simulink model "Simulator_3D2"  (R2018a)
settings: Solver=ode4  StartTime=0.0  StopTime=60  FixedStep=T  RelTol=1e-3
undefined symbols (not defined in the file): A_w, A_w2, epsilon_w, epsilon_w2, k_w, k_w2, Lc_0, omega_w, omega_w2, T, w_dir, w_dir2, zu_bar
libraries: vrlib x132
(part 1 of 6)
settings Model: Creator=Ahmad  LastModifiedBy=Ahmad

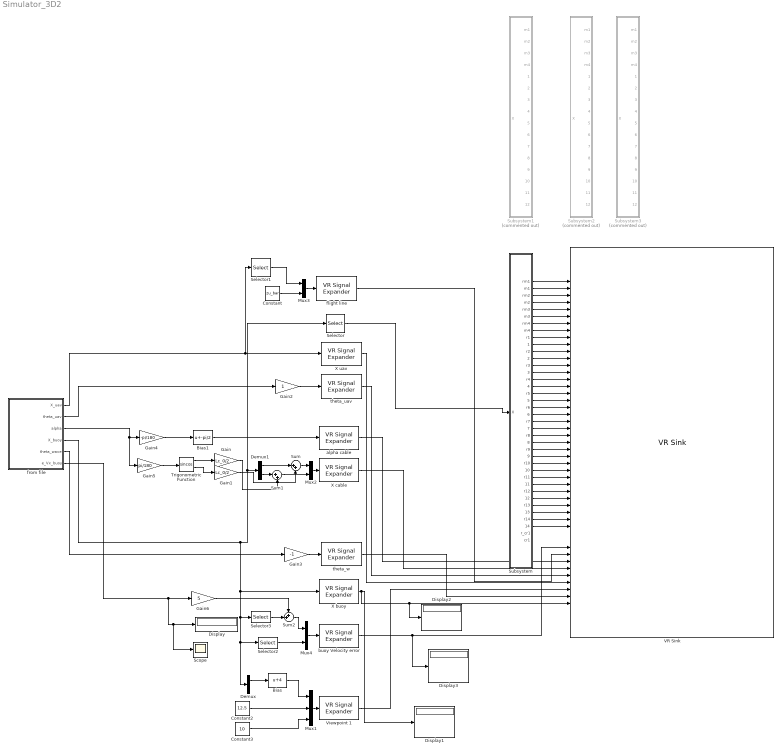
== system Simulator_3D2 ==
  Bias : Bias  Bias=4
  Bias1 : Bias  Bias=-pi/2
  Constant : Constant  Value=zu_bar
  Constant2 : Constant  Value=12.5
  Constant3 : Constant  Value=10
  Demux : Demux  Outputs=2
  Demux1 : Demux  Outputs=2
  Display{,1..3} (4 alike) : Display
  Gain : Gain  Gain=Lc_0/2
  Gain1 : Gain  Gain=Lc_0/2
  Gain2 : Gain
  Gain3 : Gain  Gain=-1
  Gain4 : Gain  Gain=-pi/180
  Gain5 : Gain  Gain=pi/180
  Gain6 : Gain  Gain=5
  Mux1 : Mux  Inputs=3
  Mux2 : Mux  Inputs=2
  Mux3 : Mux  Inputs=2
  Mux4 : Mux  Inputs=2
  Scope : Scope
  Selector : Selector  InputPortWidth=2  IndexOptions=Index vector (dialog)  Indices=[1]  OutputSizes=1
  Selector1 : Selector  InputPortWidth=2  IndexOptions=Index vector (dialog)  Indices=[1]  OutputSizes=1
  Selector2 : Selector  InputPortWidth=2  IndexOptions=Index vector (dialog)  Indices=2  OutputSizes=1
  Selector3 : Selector  InputPortWidth=2  IndexOptions=Index vector (dialog)  Indices=1  OutputSizes=1
  Subsystem : Subsystem
  Subsystem1 : Subsystem  Commented=on
  Subsystem2 : Subsystem  Commented=on
  Subsystem3 : Subsystem  Commented=on
  Sum : Sum  Inputs=|++
  Sum1 : Sum  Inputs=|++
  Sum2 : Sum  Inputs=++|
  Trigonometric Function : Trigonometry  Operator=sincos
  VR Sink : vrlib/VR Sink  InstantiateOnLoad=on  SampleTime=T  ViewEnable=on  RemoteChange=off  RemoteView=off  FieldsWritten=wave_m1.rotation.4.1.1.double#wave_m1.translation.3.1.1.double#wave_m2.rotation.4.1.1.double#wave_m2.translation.3.1.1.double#wave_m3.rotation.4.1.1.double#wave_m3.translation.3.1.1.double#wave_m4.rotation.4.1.1.double#wave_m4.translation.3.1.1.double#wave_1.rotation.4.1.1.double#wave_1.translation.3.1.1.double#wave_2.rotation.4.1.1.double#wave_2.translation.3.1.1.double#wave_3.rotation.4.1.1.double#wave_3.translation.3.1.1.double#wave_4.rotation.4.1.1.double#wave_4.translation.3.1.1.double#wave_5.rotation.4.1.1.double#wave_5.translation.3.1.1.double#wave_6.rotation.4.1.1.double#wave_6.translation.3.1.1.double#wave_7.rotation.4.1.1.double#wave_7.translation.3.1.1.double#wave_8.rotation.4.1.1.double#wave_8.translation.3.1.1.double#wave_9.rotation.4.1.1.double#wave_9.translation.3.1.1.double#wave_10.rotation.4.1.1.double#wave_10.translation.3.1.1.double#wave_11.rotation.4.1.1.double#wave_11.translation.3.1.1.double#wave_12.rotation.4.1.1.double#wave_12.translation.3.1.1.double#wave_13.rotation.4.1.1.double#wave_13.translation.3.1.1.double#wave_14.rotation.4.1.1.double#wave_14.translation.3.1.1.double#crest_1.rotation.4.1.1.double#crest_1.translation.3.1.1.double#V_ref.translation.3.1.1.double#flight_line.translation.3.1.1.double#cable.rotation.4.1.1.double#cable.translation.3.1.1.double#UAV2.rotation.4.1.1.double#UAV2.translation.3.1.1.double#Viewpoint_1_uav.position.3.1.1.double#Buoy.rotation.4.1.1.double#Buoy.translation.3.1.1.double  WorldFileName=Scene_v2.wrl  AutoView=off  VideoDimensions=[]  AllowVariableSize=off  FigureProperties="{'Position', 'Name', 'Viewpoint', 'CameraBound', 'CameraDirection', 'CameraPosition', 'CameraUpVector', 'ZoomFactor', 'Antialiasing', 'Headlight', 'Lighting', 'NavPanel', 'Sound', 'StatusBar', 'Stereo3D', 'Stereo3DCameraOffset', 'Stereo3DHIT', 'ToolBar', 'Textures', 'Transparency', 'Triad', 'Wireframe', 'NavZones', 'NavMode', 'NavSpeed', 'CaptureFileFormat', 'CaptureFileName', 'Record2DCompressMethod', 'Record2DCompressQuality', 'Record2D', 'Record2DFileName', 'Record2DFPS'; [1.8800000000000000e+02   1.7400000000000000e+02   5.7600000000000000e+02   3.5000000000000000e+02], '', '_untitled_1', 'on', [0.0000000000000000e+00   0.0000000000000000e+00  -1.0000000000000000e+00], [0.0000000000000000e+00   0.0000000000000000e+00   0.0000000000000000e+00], [0.0000000000000000e+00   1.0000000000000000e+00   0.0000000000000000e+00], [1.0000000000000000e+00], 'on', 'on', 'on', 'halfbar', 'on', 'on', 'off', [1.0000000149011612e-01], [0.0000000000000000e+00], 'on', 'on', 'on', 'none', 'off', 'off', 'fly', 'normal', 'png', '%f_anim_%n.png', 'auto', [1.0000000000000000e+02], 'on', '%f_anim_%n.avi', 'auto'}"
      settings: SourceProductBaseCode=VR
  Viewpoint 1 : vrlib/VR Signal Expander  outwidth=3  outidx=[1 2 3]
      settings: SourceProductName=Simulink 3D Animation  SourceProductBaseCode=VR
  X buoy : vrlib/VR Signal Expander  outwidth=3  outidx=[1 2]
      settings: SourceProductName=Simulink 3D Animation  SourceProductBaseCode=VR
  X cable : vrlib/VR Signal Expander  outwidth=3  outidx=[1 2]
      settings: SourceProductName=Simulink 3D Animation  SourceProductBaseCode=VR
  X uav : vrlib/VR Signal Expander  outwidth=3  outidx=[1 2]
      settings: SourceProductName=Simulink 3D Animation  SourceProductBaseCode=VR
  alpha cable : vrlib/VR Signal Expander  outwidth=4  outidx=[4]
      settings: SourceProductName=Simulink 3D Animation  SourceProductBaseCode=VR
  buoy Velocity error : vrlib/VR Signal Expander  outwidth=3  outidx=[1 2]
      settings: SourceProductName=Simulink 3D Animation  SourceProductBaseCode=VR
  flight line : vrlib/VR Signal Expander  outwidth=3  outidx=[1 2]
      settings: SourceProductName=Simulink 3D Animation  SourceProductBaseCode=VR
  from file : Subsystem
  theta_uav : vrlib/VR Signal Expander  outwidth=4  outidx=[4]
      settings: SourceProductName=Simulink 3D Animation  SourceProductBaseCode=VR
  theta_w : vrlib/VR Signal Expander  outwidth=4  outidx=[4]
      settings: SourceProductName=Simulink 3D Animation  SourceProductBaseCode=VR
  wires:
  X buoy/1 -> Display1/1, Display2/1, VR Sink/47
  Mux1/1 -> Viewpoint 1/1
  Demux/1 -> Bias/1
  Constant2/1 -> Mux1/2
  Constant3/1 -> Mux1/3
  Bias/1 -> Mux1/1
  Trigonometric Function/1 -> Gain/1
  Trigonometric Function/2 -> Gain1/1
  Demux1/1 -> Sum/1
  Mux2/1 -> X cable/1
  Sum/1 -> Mux2/1
  Demux1/2 -> Sum1/1
  Sum1/1 -> Mux2/2
  Gain1/1 -> Sum/2
  Gain/1 -> Sum1/2
  Gain2/1 -> theta_uav/1
  Gain3/1 -> theta_w/1
  Gain4/1 -> Bias1/1
  Gain5/1 -> Trigonometric Function/1
  Bias1/1 -> alpha cable/1
  Selector/1 -> Subsystem/1(X)
  Selector1/1 -> Mux3/1
  Mux3/1 -> flight line/1
  Constant/1 -> Mux3/2
  from file/3(alpha) -> Gain5/1, Gain4/1
  from file/1(X_uav) -> Selector1/1, X uav/1
  from file/4(X_buoy) -> Demux1/1, Selector/1, X buoy/1, Selector2/1, Demux/1, Selector3/1
  from file/2(theta_uav) -> Gain2/1
  from file/5(theta_wave) -> Gain3/1
  Subsystem/1(rm1) -> VR Sink/1
  Subsystem/2(m1) -> VR Sink/2
  Subsystem/3(rm2) -> VR Sink/3
  Subsystem/4(m2) -> VR Sink/4
  Subsystem/5(rm3) -> VR Sink/5
  Subsystem/6(m3) -> VR Sink/6
  Subsystem/7(rm4) -> VR Sink/7
  Subsystem/8(m4) -> VR Sink/8
  Subsystem/9(r1) -> VR Sink/9
  Subsystem/10(1) -> VR Sink/10
  Subsystem/11(r2) -> VR Sink/11
  Subsystem/12(2) -> VR Sink/12
  Subsystem/13(r3) -> VR Sink/13
  Subsystem/14(3) -> VR Sink/14
  Subsystem/15(r4) -> VR Sink/15
  Subsystem/16(4) -> VR Sink/16
  Subsystem/17(r5) -> VR Sink/17
  Subsystem/18(5) -> VR Sink/18
  Subsystem/19(r6) -> VR Sink/19
  Subsystem/20(6) -> VR Sink/20
  Subsystem/21(r7) -> VR Sink/21
  Subsystem/22(7) -> VR Sink/22
  Subsystem/23(r8) -> VR Sink/23
  Subsystem/24(8) -> VR Sink/24
  Subsystem/25(r9) -> VR Sink/25
  Subsystem/26(9) -> VR Sink/26
  Subsystem/27(r10) -> VR Sink/27
  Subsystem/28(10) -> VR Sink/28
  Subsystem/29(r11) -> VR Sink/29
  Subsystem/30(11) -> VR Sink/30
  Subsystem/31(r12) -> VR Sink/31
  Subsystem/32(12) -> VR Sink/32
  Subsystem/33(r13) -> VR Sink/33
  Subsystem/34(13) -> VR Sink/34
  Subsystem/35(r14) -> VR Sink/35
  Subsystem/36(14) -> VR Sink/36
  ? -> VR Sink/37
  ? -> VR Sink/38
  flight line/1 -> VR Sink/40
  alpha cable/1 -> VR Sink/41
  X cable/1 -> VR Sink/42
  theta_uav/1 -> VR Sink/43
  X uav/1 -> VR Sink/44
  Viewpoint 1/1 -> VR Sink/45
  theta_w/1 -> VR Sink/46
  Mux4/1 -> buoy Velocity error/1
  Selector2/1 -> Mux4/2
  Sum2/1 -> Mux4/1
  Selector3/1 -> Sum2/2
  from file/6(e_Vx_buoy) -> Scope/1, Display/1, Gain6/1
  Gain6/1 -> Sum2/1
  buoy Velocity error/1 -> Display3/1, VR Sink/39

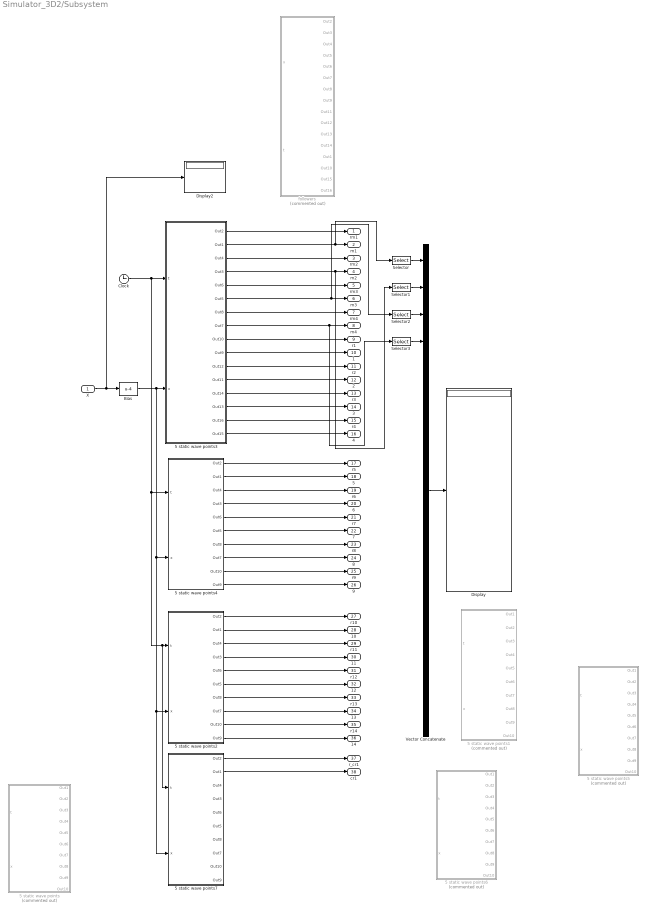
== system Simulator_3D2/Subsystem ==
  X : Inport
  5 static wave points : Subsystem  Commented=on
  5 static wave points1 : Subsystem  Commented=on
  5 static wave points2 : Subsystem
  5 static wave points3 : Subsystem
  5 static wave points4 : Subsystem
  5 static wave points5 : Subsystem  Commented=on
  5 static wave points6 : Subsystem  Commented=on
  5 static wave points7 : Subsystem
  Bias : Bias  Bias=-4
  Clock : Clock
  Display : Display
  Display2 : Display
  Selector{,1..3} (4 alike) : Selector  InputPortWidth=3  IndexOptions=Index vector (dialog)  Indices=1  OutputSizes=1
  Vector Concatenate : Concatenate  NumInputs=18
  followers : Subsystem  Commented=on
  rm1 : Outport
  m1 : Outport  Port=2
  rm2 : Outport  Port=3
  m2 : Outport  Port=4
  rm3 : Outport  Port=5
  m3 : Outport  Port=6
  rm4 : Outport  Port=7
  m4 : Outport  Port=8
  r1 : Outport  Port=9
  1 : Outport  Port=10
  r2 : Outport  Port=11
  2 : Outport  Port=12
  r3 : Outport  Port=13
  3 : Outport  Port=14
  r4 : Outport  Port=15
  4 : Outport  Port=16
  r5 : Outport  Port=17
  5 : Outport  Port=18
  r6 : Outport  Port=19
  6 : Outport  Port=20
  r7 : Outport  Port=21
  7 : Outport  Port=22
  r8 : Outport  Port=23
  8 : Outport  Port=24
  r9 : Outport  Port=25
  9 : Outport  Port=26
  r10 : Outport  Port=27
  10 : Outport  Port=28
  r11 : Outport  Port=29
  11 : Outport  Port=30
  r12 : Outport  Port=31
  12 : Outport  Port=32
  r13 : Outport  Port=33
  13 : Outport  Port=34
  r14 : Outport  Port=35
  14 : Outport  Port=36
  r_cr1 : Outport  Port=37
  cr1 : Outport  Port=38
  wires:
  X/1 -> Bias/1, Display2/1
  5 static wave points4/9(Out10) -> r9/1
  5 static wave points3/12(Out11) -> 2/1
  5 static wave points3/6(Out5) -> Selector2/1, m3/1
  5 static wave points3/10(Out9) -> 1/1
  5 static wave points3/8(Out7) -> Selector3/1, m4/1
  5 static wave points4/1(Out2) -> r5/1
  5 static wave points4/3(Out4) -> r6/1
  5 static wave points4/5(Out6) -> r7/1
  5 static wave points4/7(Out8) -> r8/1
  5 static wave points2/1(Out2) -> r10/1
  5 static wave points3/4(Out3) -> Selector1/1, m2/1
  Clock/1 -> 5 static wave points3/1(t), 5 static wave points7/1(t), 5 static wave points2/1(t), 5 static wave points4/1(t)
  Bias/1 -> 5 static wave points7/2(x), 5 static wave points2/2(x), 5 static wave points4/2(x), 5 static wave points3/2(x)
  5 static wave points3/3(Out4) -> rm2/1
  5 static wave points3/5(Out6) -> rm3/1
  5 static wave points3/1(Out2) -> rm1/1
  5 static wave points3/7(Out8) -> rm4/1
  5 static wave points3/9(Out10) -> r1/1
  5 static wave points3/11(Out12) -> r2/1
  5 static wave points4/2(Out1) -> 5/1
  5 static wave points4/4(Out3) -> 6/1
  5 static wave points4/6(Out5) -> 7/1
  5 static wave points4/10(Out9) -> 9/1
  5 static wave points4/8(Out7) -> 8/1
  5 static wave points2/2(Out1) -> 10/1
  5 static wave points2/3(Out4) -> r11/1
  5 static wave points2/4(Out3) -> 11/1
  5 static wave points2/5(Out6) -> r12/1
  5 static wave points2/6(Out5) -> 12/1
  5 static wave points2/10(Out9) -> 14/1
  5 static wave points2/9(Out10) -> r14/1
  5 static wave points2/8(Out7) -> 13/1
  5 static wave points2/7(Out8) -> r13/1
  5 static wave points3/2(Out1) -> Selector/1, m1/1
  Vector Concatenate/1 -> Display/1
  Selector/1 -> Vector Concatenate/1
  Selector1/1 -> Vector Concatenate/2
  Selector2/1 -> Vector Concatenate/3
  Selector3/1 -> Vector Concatenate/4
  5 static wave points3/13(Out14) -> r3/1
  5 static wave points3/14(Out13) -> 3/1
  5 static wave points3/15(Out16) -> r4/1
  5 static wave points3/16(Out15) -> 4/1
  5 static wave points7/1(Out2) -> r_cr1/1
  5 static wave points7/2(Out1) -> cr1/1

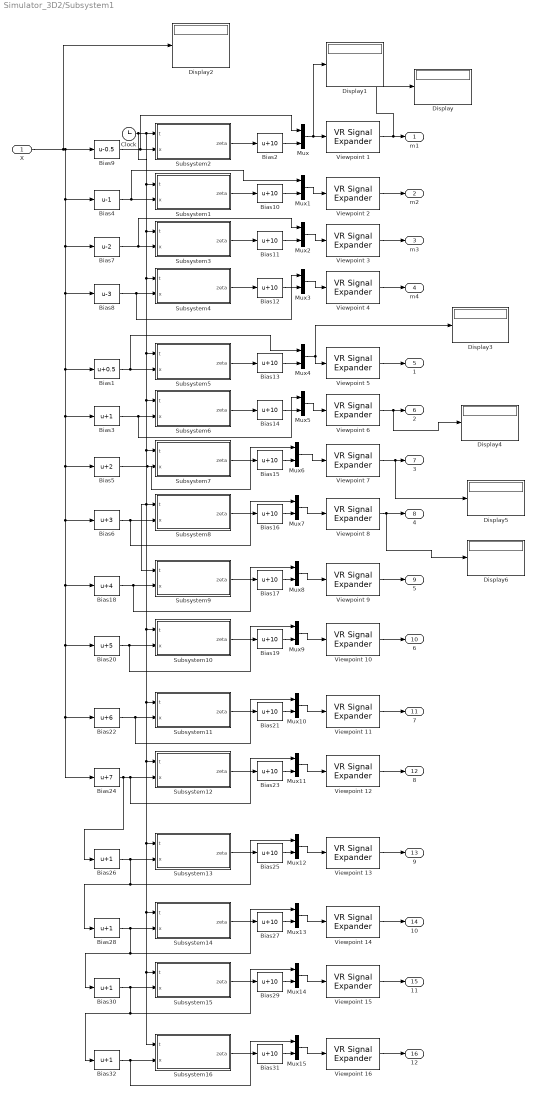
== system Simulator_3D2/Subsystem1 ==
  X : Inport
  Bias1 : Bias  Bias=0.5
  Bias{2,10..17,19,21,23,25,27,29,31} (16 alike) : Bias  Bias=10
  Bias18 : Bias  Bias=4
  Bias20 : Bias  Bias=5
  Bias22 : Bias  Bias=6
  Bias24 : Bias  Bias=7
  Bias{3,26,28,30,32} (5 alike) : Bias  Bias=1
  Bias4 : Bias  Bias=-1
  Bias5 : Bias  Bias=2
  Bias6 : Bias  Bias=3
  Bias7 : Bias  Bias=-2
  Bias8 : Bias  Bias=-3
  Bias9 : Bias  Bias=-0.5
  Clock : Clock
  Display{,1..6} (7 alike) : Display
  Mux{,1..15} (16 alike) : Mux  Inputs=2
  Subsystem1 : Subsystem
  Subsystem10 : Subsystem
  Subsystem11 : Subsystem
  Subsystem12 : Subsystem
  Subsystem13 : Subsystem
  Subsystem14 : Subsystem
  Subsystem15 : Subsystem
  Subsystem16 : Subsystem
  Subsystem2 : Subsystem
  Subsystem3 : Subsystem
  Subsystem4 : Subsystem
  Subsystem5 : Subsystem
  Subsystem6 : Subsystem
  Subsystem7 : Subsystem
  Subsystem8 : Subsystem
  Subsystem9 : Subsystem
  Viewpoint {1..16} (16 alike) : vrlib/VR Signal Expander  outwidth=3  outidx=[1 2]
      settings: SourceProductName=Simulink 3D Animation  SourceProductBaseCode=VR
  m1 : Outport
  m2 : Outport  Port=2
  m3 : Outport  Port=3
  m4 : Outport  Port=4
  1 : Outport  Port=5
  2 : Outport  Port=6
  3 : Outport  Port=7
  4 : Outport  Port=8
  5 : Outport  Port=9
  6 : Outport  Port=10
  7 : Outport  Port=11
  8 : Outport  Port=12
  9 : Outport  Port=13
  10 : Outport  Port=14
  11 : Outport  Port=15
  12 : Outport  Port=16
  wires:
  Subsystem2/1(zeta) -> Bias2/1
  Bias9/1 -> Subsystem2/2(x), Mux/1
  Bias8/1 -> Subsystem4/2(x), Mux3/1
  Bias4/1 -> Subsystem1/2(x), Mux1/1
  Subsystem1/1(zeta) -> Bias10/1
  Subsystem3/1(zeta) -> Bias11/1
  Subsystem4/1(zeta) -> Bias12/1
  Subsystem5/1(zeta) -> Bias13/1
  Subsystem6/1(zeta) -> Bias14/1
  Subsystem7/1(zeta) -> Bias15/1
  Subsystem8/1(zeta) -> Bias16/1
  Bias3/1 -> Subsystem6/2(x), Mux5/1
  Bias6/1 -> Subsystem8/2(x), Mux7/1
  Viewpoint 1/1 -> Display/1, m1/1
  Viewpoint 2/1 -> m2/1
  Viewpoint 3/1 -> m3/1
  Viewpoint 4/1 -> m4/1
  Viewpoint 5/1 -> 1/1
  Viewpoint 6/1 -> Display4/1, 2/1
  Viewpoint 8/1 -> Display6/1, 4/1
  Mux/1 -> Display1/1, Viewpoint 1/1
  Mux1/1 -> Viewpoint 2/1
  Mux2/1 -> Viewpoint 3/1
  Mux3/1 -> Viewpoint 4/1
  Mux4/1 -> Display3/1, Viewpoint 5/1
  Mux5/1 -> Viewpoint 6/1
  Mux6/1 -> Viewpoint 7/1
  Mux7/1 -> Viewpoint 8/1
  Bias2/1 -> Mux/2
  Bias10/1 -> Mux1/2
  Bias11/1 -> Mux2/2
  Bias7/1 -> Subsystem3/2(x), Mux2/1
  Bias12/1 -> Mux3/2
  Bias13/1 -> Mux4/2
  Bias1/1 -> Subsystem5/2(x), Mux4/1
  Bias14/1 -> Mux5/2
  Bias15/1 -> Mux6/2
  Bias5/1 -> Mux6/1, Subsystem7/2(x)
  Bias16/1 -> Mux7/2
  Bias17/1 -> Mux8/2
  Mux8/1 -> Viewpoint 9/1
  Viewpoint 9/1 -> 5/1
  Bias18/1 -> Subsystem9/2(x), Mux8/1
  Subsystem9/1(zeta) -> Bias17/1
  Subsystem10/1(zeta) -> Bias19/1
  Bias20/1 -> Subsystem10/2(x), Mux9/1
  Viewpoint 10/1 -> 6/1
  Mux9/1 -> Viewpoint 10/1
  Bias19/1 -> Mux9/2
  Bias21/1 -> Mux10/2
  Mux10/1 -> Viewpoint 11/1
  Viewpoint 11/1 -> 7/1
  Bias22/1 -> Subsystem11/2(x), Mux10/1
  Subsystem11/1(zeta) -> Bias21/1
  Subsystem12/1(zeta) -> Bias23/1
  Bias24/1 -> Bias26/1, Subsystem12/2(x), Mux11/1
  Viewpoint 12/1 -> 8/1
  Mux11/1 -> Viewpoint 12/1
  Bias23/1 -> Mux11/2
  Viewpoint 7/1 -> Display5/1, 3/1
  Bias25/1 -> Mux12/2
  Mux12/1 -> Viewpoint 13/1
  Viewpoint 13/1 -> 9/1
  Bias26/1 -> Bias28/1, Mux12/1, Subsystem13/2(x)
  Subsystem13/1(zeta) -> Bias25/1
  X/1 -> Display2/1, Bias4/1, Bias7/1, Bias24/1, Bias22/1, Bias20/1, Bias18/1, Bias6/1, Bias5/1, Bias3/1, Bias1/1, Bias8/1, Bias9/1
  Subsystem14/1(zeta) -> Bias27/1
  Bias28/1 -> Subsystem14/2(x), Bias30/1, Mux13/1
  Viewpoint 14/1 -> 10/1
  Mux13/1 -> Viewpoint 14/1
  Bias27/1 -> Mux13/2
  Bias29/1 -> Mux14/2
  Mux14/1 -> Viewpoint 15/1
  Viewpoint 15/1 -> 11/1
  Bias30/1 -> Bias32/1, Mux14/1, Subsystem15/2(x)
  Subsystem15/1(zeta) -> Bias29/1
  Clock/1 -> Subsystem9/1(t), Subsystem8/1(t), Subsystem7/1(t), Subsystem6/1(t), Subsystem5/1(t), Subsystem4/1(t), Subsystem3/1(t), Subsystem1/1(t), Subsystem2/1(t), Subsystem11/1(t), Subsystem16/1(t), Subsystem15/1(t), Subsystem14/1(t), Subsystem13/1(t), Subsystem12/1(t), Subsystem10/1(t)
  Subsystem16/1(zeta) -> Bias31/1
  Bias32/1 -> Subsystem16/2(x), Mux15/1
  Viewpoint 16/1 -> 12/1
  Mux15/1 -> Viewpoint 16/1
  Bias31/1 -> Mux15/2

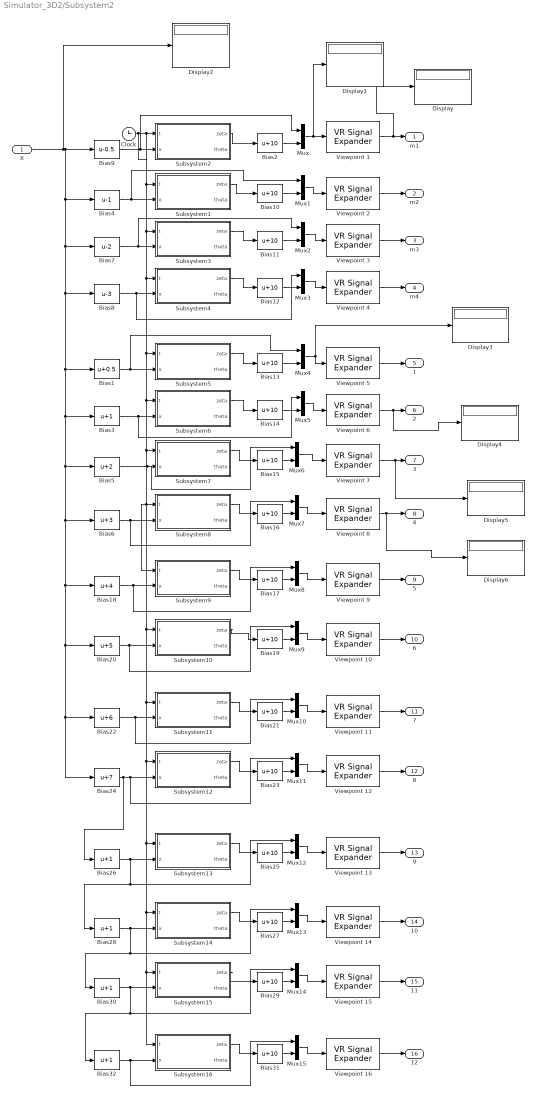
== system Simulator_3D2/Subsystem2 ==
  X : Inport
  Bias1 : Bias  Bias=0.5
  Bias{2,10..17,19,21,23,25,27,29,31} (16 alike) : Bias  Bias=10
  Bias18 : Bias  Bias=4
  Bias20 : Bias  Bias=5
  Bias22 : Bias  Bias=6
  Bias24 : Bias  Bias=7
  Bias{3,26,28,30,32} (5 alike) : Bias  Bias=1
  Bias4 : Bias  Bias=-1
  Bias5 : Bias  Bias=2
  Bias6 : Bias  Bias=3
  Bias7 : Bias  Bias=-2
  Bias8 : Bias  Bias=-3
  Bias9 : Bias  Bias=-0.5
  Clock : Clock
  Display{,1..6} (7 alike) : Display
  Mux{,1..15} (16 alike) : Mux  Inputs=2
  Subsystem1 : Subsystem
  Subsystem10 : Subsystem
  Subsystem11 : Subsystem
  Subsystem12 : Subsystem
  Subsystem13 : Subsystem
  Subsystem14 : Subsystem
  Subsystem15 : Subsystem
  Subsystem16 : Subsystem
  Subsystem2 : Subsystem
  Subsystem3 : Subsystem
  Subsystem4 : Subsystem
  Subsystem5 : Subsystem
  Subsystem6 : Subsystem
  Subsystem7 : Subsystem
  Subsystem8 : Subsystem
  Subsystem9 : Subsystem
  Viewpoint {1..16} (16 alike) : vrlib/VR Signal Expander  outwidth=3  outidx=[1 2]
      settings: SourceProductName=Simulink 3D Animation  SourceProductBaseCode=VR
  m1 : Outport
  m2 : Outport  Port=2
  m3 : Outport  Port=3
  m4 : Outport  Port=4
  1 : Outport  Port=5
  2 : Outport  Port=6
  3 : Outport  Port=7
  4 : Outport  Port=8
  5 : Outport  Port=9
  6 : Outport  Port=10
  7 : Outport  Port=11
  8 : Outport  Port=12
  9 : Outport  Port=13
  10 : Outport  Port=14
  11 : Outport  Port=15
  12 : Outport  Port=16
  wires:
  Subsystem2/1(zeta) -> Bias2/1
  Bias9/1 -> Subsystem2/2(x), Mux/1
  Bias8/1 -> Subsystem4/2(x), Mux3/1
  Bias4/1 -> Subsystem1/2(x), Mux1/1
  Subsystem8/1(zeta) -> Bias16/1
  Bias3/1 -> Subsystem6/2(x), Mux5/1
  Bias6/1 -> Subsystem8/2(x), Mux7/1
  Viewpoint 1/1 -> Display/1, m1/1
  Viewpoint 2/1 -> m2/1
  Viewpoint 3/1 -> m3/1
  Viewpoint 4/1 -> m4/1
  Viewpoint 5/1 -> 1/1
  Viewpoint 6/1 -> Display4/1, 2/1
  Viewpoint 8/1 -> Display6/1, 4/1
  Mux/1 -> Display1/1, Viewpoint 1/1
  Mux1/1 -> Viewpoint 2/1
  Mux2/1 -> Viewpoint 3/1
  Mux3/1 -> Viewpoint 4/1
  Mux4/1 -> Display3/1, Viewpoint 5/1
  Mux5/1 -> Viewpoint 6/1
  Mux6/1 -> Viewpoint 7/1
  Mux7/1 -> Viewpoint 8/1
  Bias2/1 -> Mux/2
  Bias10/1 -> Mux1/2
  Bias11/1 -> Mux2/2
  Bias7/1 -> Subsystem3/2(x), Mux2/1
  Bias12/1 -> Mux3/2
  Bias13/1 -> Mux4/2
  Bias1/1 -> Subsystem5/2(x), Mux4/1
  Bias14/1 -> Mux5/2
  Bias15/1 -> Mux6/2
  Bias5/1 -> Mux6/1, Subsystem7/2(x)
  Bias16/1 -> Mux7/2
  Bias17/1 -> Mux8/2
  Mux8/1 -> Viewpoint 9/1
  Viewpoint 9/1 -> 5/1
  Bias18/1 -> Subsystem9/2(x), Mux8/1
  Subsystem10/1(zeta) -> Bias19/1
  Bias20/1 -> Subsystem10/2(x), Mux9/1
  Viewpoint 10/1 -> 6/1
  Mux9/1 -> Viewpoint 10/1
  Bias19/1 -> Mux9/2
  Bias21/1 -> Mux10/2
  Mux10/1 -> Viewpoint 11/1
  Viewpoint 11/1 -> 7/1
  Bias22/1 -> Subsystem11/2(x), Mux10/1
  Subsystem11/1(zeta) -> Bias21/1
  Bias24/1 -> Bias26/1, Subsystem12/2(x), Mux11/1
  Viewpoint 12/1 -> 8/1
  Mux11/1 -> Viewpoint 12/1
  Bias23/1 -> Mux11/2
  Viewpoint 7/1 -> Display5/1, 3/1
  Bias25/1 -> Mux12/2
  Mux12/1 -> Viewpoint 13/1
  Viewpoint 13/1 -> 9/1
  Bias26/1 -> Subsystem13/2(x), Bias28/1, Mux12/1
  X/1 -> Display2/1, Bias4/1, Bias7/1, Bias24/1, Bias22/1, Bias20/1, Bias18/1, Bias6/1, Bias5/1, Bias3/1, Bias1/1, Bias8/1, Bias9/1
  Bias28/1 -> Subsystem14/2(x), Bias30/1, Mux13/1
  Viewpoint 14/1 -> 10/1
  Mux13/1 -> Viewpoint 14/1
  Bias27/1 -> Mux13/2
  Bias29/1 -> Mux14/2
  Mux14/1 -> Viewpoint 15/1
  Viewpoint 15/1 -> 11/1
  Bias30/1 -> Subsystem15/2(x), Bias32/1, Mux14/1
  Subsystem15/1(zeta) -> Bias29/1
  Clock/1 -> Subsystem1/1(t), Subsystem3/1(t), Subsystem4/1(t), Subsystem5/1(t), Subsystem6/1(t), Subsystem7/1(t), Subsystem9/1(t), Subsystem8/1(t), Subsystem2/1(t), Subsystem10/1(t), Subsystem11/1(t), Subsystem12/1(t), Subsystem13/1(t), Subsystem14/1(t), Subsystem16/1(t), Subsystem15/1(t)
  Subsystem16/1(zeta) -> Bias31/1
  Bias32/1 -> Subsystem16/2(x), Mux15/1
  Viewpoint 16/1 -> 12/1
  Mux15/1 -> Viewpoint 16/1
  Bias31/1 -> Mux15/2
  Subsystem7/1(zeta) -> Bias15/1
  Subsystem14/1(zeta) -> Bias27/1
  Subsystem13/1(zeta) -> Bias25/1
  Subsystem12/1(zeta) -> Bias23/1
  Subsystem9/1(zeta) -> Bias17/1
  Subsystem6/1(zeta) -> Bias14/1
  Subsystem5/1(zeta) -> Bias13/1
  Subsystem4/1(zeta) -> Bias12/1
  Subsystem3/1(zeta) -> Bias11/1
  Subsystem1/1(zeta) -> Bias10/1

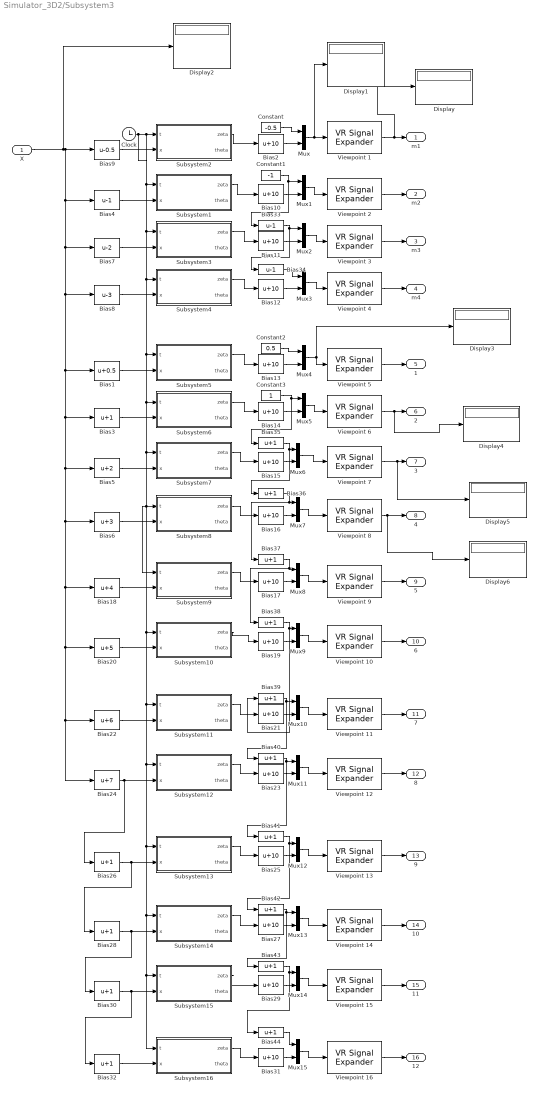
== system Simulator_3D2/Subsystem3 ==
  X : Inport
  Bias1 : Bias  Bias=0.5
  Bias{2,10..17,19,21,23,25,27,29,31} (16 alike) : Bias  Bias=10
  Bias18 : Bias  Bias=4
  Bias20 : Bias  Bias=5
  Bias22 : Bias  Bias=6
  Bias24 : Bias  Bias=7
  Bias{3,26,28,30,32,35..44} (15 alike) : Bias  Bias=1
  Bias33 : Bias  Bias=-1
  Bias34 : Bias  Bias=-1
  Bias4 : Bias  Bias=-1
  Bias5 : Bias  Bias=2
  Bias6 : Bias  Bias=3
  Bias7 : Bias  Bias=-2
  Bias8 : Bias  Bias=-3
  Bias9 : Bias  Bias=-0.5
  Clock : Clock
  Constant : Constant  Value=-0.5
  Constant1 : Constant  Value=-1
  Constant2 : Constant  Value=0.5
  Constant3 : Constant
  Display{,1..6} (7 alike) : Display
  Mux{,1..15} (16 alike) : Mux  Inputs=2
  Subsystem1 : Subsystem
  Subsystem10 : Subsystem
  Subsystem11 : Subsystem
  Subsystem12 : Subsystem
  Subsystem13 : Subsystem
  Subsystem14 : Subsystem
  Subsystem15 : Subsystem
  Subsystem16 : Subsystem
  Subsystem2 : Subsystem
  Subsystem3 : Subsystem
  Subsystem4 : Subsystem
  Subsystem5 : Subsystem
  Subsystem6 : Subsystem
  Subsystem7 : Subsystem
  Subsystem8 : Subsystem
  Subsystem9 : Subsystem
  Viewpoint {1..16} (16 alike) : vrlib/VR Signal Expander  outwidth=3  outidx=[1 2]
      settings: SourceProductName=Simulink 3D Animation  SourceProductBaseCode=VR
  m1 : Outport
  m2 : Outport  Port=2
  m3 : Outport  Port=3
  m4 : Outport  Port=4
  1 : Outport  Port=5
  2 : Outport  Port=6
  3 : Outport  Port=7
  4 : Outport  Port=8
  5 : Outport  Port=9
  6 : Outport  Port=10
  7 : Outport  Port=11
  8 : Outport  Port=12
  9 : Outport  Port=13
  10 : Outport  Port=14
  11 : Outport  Port=15
  12 : Outport  Port=16
  wires:
  Subsystem2/1(zeta) -> Bias2/1
  Bias9/1 -> Subsystem2/2(x)
  Bias8/1 -> Subsystem4/2(x)
  Bias4/1 -> Subsystem1/2(x)
  Subsystem8/1(zeta) -> Bias16/1
  Bias3/1 -> Subsystem6/2(x)
  Bias6/1 -> Subsystem8/2(x)
  Viewpoint 1/1 -> Display/1, m1/1
  Viewpoint 2/1 -> m2/1
  Viewpoint 3/1 -> m3/1
  Viewpoint 4/1 -> m4/1
  Viewpoint 5/1 -> 1/1
  Viewpoint 6/1 -> Display4/1, 2/1
  Viewpoint 8/1 -> Display6/1, 4/1
  Mux/1 -> Display1/1, Viewpoint 1/1
  Mux1/1 -> Viewpoint 2/1
  Mux2/1 -> Viewpoint 3/1
  Mux3/1 -> Viewpoint 4/1
  Mux4/1 -> Display3/1, Viewpoint 5/1
  Mux5/1 -> Viewpoint 6/1
  Mux6/1 -> Viewpoint 7/1
  Mux7/1 -> Viewpoint 8/1
  Bias2/1 -> Mux/2
  Bias10/1 -> Mux1/2
  Bias11/1 -> Mux2/2
  Bias7/1 -> Subsystem3/2(x)
  Bias12/1 -> Mux3/2
  Bias13/1 -> Mux4/2
  Bias1/1 -> Subsystem5/2(x)
  Bias14/1 -> Mux5/2
  Bias15/1 -> Mux6/2
  Bias5/1 -> Subsystem7/2(x)
  Bias16/1 -> Mux7/2
  Bias17/1 -> Mux8/2
  Mux8/1 -> Viewpoint 9/1
  Viewpoint 9/1 -> 5/1
  Bias18/1 -> Subsystem9/2(x)
  Subsystem10/1(zeta) -> Bias19/1
  Bias20/1 -> Subsystem10/2(x)
  Viewpoint 10/1 -> 6/1
  Mux9/1 -> Viewpoint 10/1
  Bias19/1 -> Mux9/2
  Bias21/1 -> Mux10/2
  Mux10/1 -> Viewpoint 11/1
  Viewpoint 11/1 -> 7/1
  Bias22/1 -> Subsystem11/2(x)
  Subsystem11/1(zeta) -> Bias21/1
  Bias24/1 -> Bias26/1, Subsystem12/2(x)
  Viewpoint 12/1 -> 8/1
  Mux11/1 -> Viewpoint 12/1
  Bias23/1 -> Mux11/2
  Viewpoint 7/1 -> Display5/1, 3/1
  Bias25/1 -> Mux12/2
  Mux12/1 -> Viewpoint 13/1
  Viewpoint 13/1 -> 9/1
  Bias26/1 -> Subsystem13/2(x), Bias28/1
  X/1 -> Display2/1, Bias4/1, Bias7/1, Bias24/1, Bias22/1, Bias20/1, Bias18/1, Bias6/1, Bias5/1, Bias3/1, Bias1/1, Bias8/1, Bias9/1
  Bias28/1 -> Subsystem14/2(x), Bias30/1
  Viewpoint 14/1 -> 10/1
  Mux13/1 -> Viewpoint 14/1
  Bias27/1 -> Mux13/2
  Bias29/1 -> Mux14/2
  Mux14/1 -> Viewpoint 15/1
  Viewpoint 15/1 -> 11/1
  Bias30/1 -> Subsystem15/2(x), Bias32/1
  Subsystem15/1(zeta) -> Bias29/1
  Clock/1 -> Subsystem1/1(t), Subsystem3/1(t), Subsystem4/1(t), Subsystem5/1(t), Subsystem6/1(t), Subsystem7/1(t), Subsystem9/1(t), Subsystem8/1(t), Subsystem2/1(t), Subsystem10/1(t), Subsystem11/1(t), Subsystem12/1(t), Subsystem13/1(t), Subsystem14/1(t), Subsystem16/1(t), Subsystem15/1(t)
  Subsystem16/1(zeta) -> Bias31/1
  Bias32/1 -> Subsystem16/2(x)
  Viewpoint 16/1 -> 12/1
  Mux15/1 -> Viewpoint 16/1
  Bias31/1 -> Mux15/2
  Subsystem7/1(zeta) -> Bias15/1
  Subsystem14/1(zeta) -> Bias27/1
  Subsystem13/1(zeta) -> Bias25/1
  Subsystem12/1(zeta) -> Bias23/1
  Subsystem9/1(zeta) -> Bias17/1
  Subsystem6/1(zeta) -> Bias14/1
  Subsystem5/1(zeta) -> Bias13/1
  Subsystem4/1(zeta) -> Bias12/1
  Subsystem3/1(zeta) -> Bias11/1
  Subsystem1/1(zeta) -> Bias10/1
  Constant/1 -> Mux/1
  Constant1/1 -> Bias33/1, Mux1/1
  Bias33/1 -> Bias34/1, Mux2/1
  Bias34/1 -> Mux3/1
  Constant2/1 -> Mux4/1
  Constant3/1 -> Bias35/1, Mux5/1
  Bias35/1 -> Bias36/1, Mux6/1
  Bias36/1 -> Bias37/1, Mux7/1
  Bias37/1 -> Bias38/1, Mux8/1
  Bias38/1 -> Bias39/1, Mux9/1
  Bias39/1 -> Bias40/1, Mux10/1
  Bias40/1 -> Bias41/1, Mux11/1
  Bias41/1 -> Bias42/1, Mux12/1
  Bias42/1 -> Bias43/1, Mux13/1
  Bias43/1 -> Bias44/1, Mux14/1
  Bias44/1 -> Mux15/1

== system Simulator_3D2/from file ==
  From File : FromFile  FileName=Export/Wavy/Lyapunov/X_b.mat  SampleTime=0
  From File1 : FromFile  FileName=Export/Wavy/Lyapunov/X_q.mat  SampleTime=0
  From File10 : FromFile  FileName=Export/Wavy/Lyapunov/V_bar.mat  SampleTime=0
  From File11 : FromFile  FileName=Export/Wavy/PID/V_bar.mat  SampleTime=0
  From File12 : FromFile  FileName=Export/Wavy/Lyapunov/Xdot_b.mat  SampleTime=0
  From File13 : FromFile  FileName=Export/Wavy/PID/Xdot_b.mat  SampleTime=0
  From File14 : FromFile  FileName=Export/No waves/Lyapunov/X_q.mat  SampleTime=0
  From File15 : FromFile  FileName=Export/No waves/PID/X_q.mat  SampleTime=0
  From File16 : FromFile  FileName=Export/No waves/Lyapunov/theta_q.mat  SampleTime=0
  From File17 : FromFile  FileName=Export/No waves/PID/theta_q.mat  SampleTime=0
  From File18 : FromFile  FileName=Export/No waves/Lyapunov/alpha.mat  SampleTime=0
  From File19 : FromFile  FileName=Export/No waves/PID/alpha.mat  SampleTime=0
  From File2 : FromFile  FileName=Export/Wavy/Lyapunov/alpha.mat  SampleTime=0
  From File20 : FromFile  FileName=Export/No waves/Lyapunov/theta_w.mat  SampleTime=0
  From File21 : FromFile  FileName=Export/No waves/PID/theta_w.mat  SampleTime=0
  From File22 : FromFile  FileName=Export/No waves/Lyapunov/X_b.mat  SampleTime=0
  From File23 : FromFile  FileName=Export/No waves/PID/X_b.mat  SampleTime=0
  From File24 : FromFile  FileName=Export/No waves/Lyapunov/V_bar.mat  SampleTime=0
  From File25 : FromFile  FileName=Export/No waves/PID/V_bar.mat  SampleTime=0
  From File26 : FromFile  FileName=Export/No waves/Lyapunov/Xdot_b.mat  SampleTime=0
  From File27 : FromFile  FileName=Export/No waves/PID/Xdot_b.mat  SampleTime=0
  From File3 : FromFile  FileName=Export/Wavy/Lyapunov/theta_q.mat  SampleTime=0
  From File4 : FromFile  FileName=Export/Wavy/Lyapunov/theta_w.mat  SampleTime=0
  From File5 : FromFile  FileName=Export/Wavy/PID/X_q.mat  SampleTime=0
  From File6 : FromFile  FileName=Export/Wavy/PID/theta_q.mat  SampleTime=0
  From File7 : FromFile  FileName=Export/Wavy/PID/alpha.mat  SampleTime=0
  From File8 : FromFile  FileName=Export/Wavy/PID/theta_w.mat  SampleTime=0
  From File9 : FromFile  FileName=Export/Wavy/PID/X_b.mat  SampleTime=0
  Selector3 : Selector  InputPortWidth=2  IndexOptions=Index vector (dialog)  Indices=1  OutputSizes=1
  Sum : Sum  Inputs=|+-
  X_uav : Outport
  theta_uav : Outport  Port=2
  alpha : Outport  Port=3
  X_buoy : Outport  Port=4
  theta_wave : Outport  Port=5
  e_Vx_buoy : Outport  Port=6
  wires:
  From File21/1 -> theta_wave/1
  From File15/1 -> X_uav/1
  From File17/1 -> theta_uav/1
  From File19/1 -> alpha/1
  From File23/1 -> X_buoy/1
  Sum/1 -> e_Vx_buoy/1
  From File25/1 -> Sum/1
  From File27/1 -> Selector3/1
  Selector3/1 -> Sum/2

== system Simulator_3D2/Subsystem/5 static wave points ==
  t : Inport
  x : Inport  Port=2
  Bias{23..32} (10 alike) : Bias  Bias=10
  Mux{11..15} (5 alike) : Mux  Inputs=2
  Subsystem12 : Subsystem
  Subsystem13 : Subsystem
  Subsystem14 : Subsystem
  Subsystem15 : Subsystem
  Subsystem16 : Subsystem
  Viewpoint {12..16} (5 alike) : vrlib/VR Signal Expander  outwidth=3  outidx=[1 2]
      settings: SourceProductName=Simulink 3D Animation  SourceProductBaseCode=VR
  Out1 : Outport
  Out2 : Outport  Port=2
  Out3 : Outport  Port=3
  Out4 : Outport  Port=4
  Out5 : Outport  Port=5
  Out6 : Outport  Port=6
  Out7 : Outport  Port=7
  Out8 : Outport  Port=8
  Out9 : Outport  Port=9
  Out10 : Outport  Port=10
  wires:
  t/1 -> Subsystem12/1(t), Subsystem13/1(t), Subsystem14/1(t), Subsystem16/1(t), Subsystem15/1(t)
  Subsystem15/1(zeta) -> Bias29/1
  Viewpoint 15/1 -> Out7/1
  Subsystem12/1(zeta) -> Bias23/1
  Viewpoint 12/1 -> Out1/1
  Mux14/1 -> Viewpoint 15/1
  Bias24/1 -> Bias26/1, Mux11/1, Subsystem12/2(x)
  Bias29/1 -> Mux14/2
  Subsystem16/1(zeta) -> Bias31/1
  Subsystem12/2(theta) -> Out2/1
  Bias32/1 -> Mux15/1, Subsystem16/2(x)
  Viewpoint 16/1 -> Out9/1
  Bias31/1 -> Mux15/2
  Mux15/1 -> Viewpoint 16/1
  x/1 -> Bias24/1
  Subsystem15/2(theta) -> Out8/1
  Bias25/1 -> Mux12/2
  Subsystem14/1(zeta) -> Bias27/1
  Mux11/1 -> Viewpoint 12/1
  Bias23/1 -> Mux11/2
  Mux12/1 -> Viewpoint 13/1
  Subsystem16/2(theta) -> Out10/1
  Subsystem13/1(zeta) -> Bias25/1
  Mux13/1 -> Viewpoint 14/1
  Viewpoint 14/1 -> Out5/1
  Bias27/1 -> Mux13/2
  Subsystem13/2(theta) -> Out4/1
  Viewpoint 13/1 -> Out3/1
  Subsystem14/2(theta) -> Out6/1
  Bias28/1 -> Mux13/1, Subsystem14/2(x), Bias30/1
  Bias26/1 -> Mux12/1, Subsystem13/2(x), Bias28/1
  Bias30/1 -> Mux14/1, Subsystem15/2(x), Bias32/1

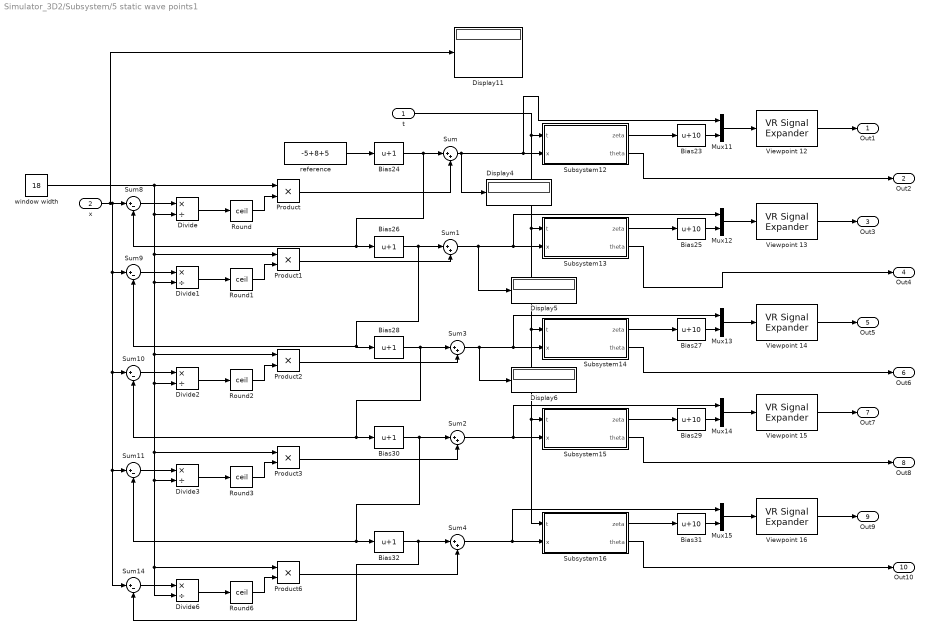
== system Simulator_3D2/Subsystem/5 static wave points1 ==
  t : Inport
  x : Inport  Port=2
  Bias{23,25,27,29,31} (5 alike) : Bias  Bias=10
  Bias{24,26,28,30,32} (5 alike) : Bias  Bias=1
  Display{4..6,11} (4 alike) : Display
  Divide{,1..3,6} (5 alike) : Product  Inputs=*/
  Mux{11..15} (5 alike) : Mux  Inputs=2
  Product{,1..3,6} (5 alike) : Product
  Round{,1..3,6} (5 alike) : Rounding  Operator=ceil
  Subsystem12 : Subsystem
  Subsystem13 : Subsystem
  Subsystem14 : Subsystem
  Subsystem15 : Subsystem
  Subsystem16 : Subsystem
  Sum{,1..4} (5 alike) : Sum  Inputs=|++
  Sum{8..11,14} (5 alike) : Sum  Inputs=|+-
  Viewpoint {12..16} (5 alike) : vrlib/VR Signal Expander  outwidth=3  outidx=[1 2]
      settings: SourceProductName=Simulink 3D Animation  SourceProductBaseCode=VR
  reference : Constant  Value=-5+8+5
  window width : Constant  Value=18
  Out1 : Outport
  Out2 : Outport  Port=2
  Out3 : Outport  Port=3
  Out4 : Outport  Port=4
  Out5 : Outport  Port=5
  Out6 : Outport  Port=6
  Out7 : Outport  Port=7
  Out8 : Outport  Port=8
  Out9 : Outport  Port=9
  Out10 : Outport  Port=10
  wires:
  reference/1 -> Bias24/1
  Sum8/1 -> Divide/1
  Divide/1 -> Round/1
  Round/1 -> Product/2
  Subsystem15/1(zeta) -> Bias29/1
  Viewpoint 15/1 -> Out7/1
  Subsystem12/1(zeta) -> Bias23/1
  Viewpoint 12/1 -> Out1/1
  Mux14/1 -> Viewpoint 15/1
  Sum/1 -> Display4/1, Mux11/1, Subsystem12/2(x)
  Bias29/1 -> Mux14/2
  Subsystem16/1(zeta) -> Bias31/1
  Subsystem12/2(theta) -> Out2/1
  Sum4/1 -> Mux15/1, Subsystem16/2(x)
  Viewpoint 16/1 -> Out9/1
  Bias31/1 -> Mux15/2
  Mux15/1 -> Viewpoint 16/1
  Subsystem15/2(theta) -> Out8/1
  Bias25/1 -> Mux12/2
  Subsystem14/1(zeta) -> Bias27/1
  Mux11/1 -> Viewpoint 12/1
  Bias23/1 -> Mux11/2
  Mux12/1 -> Viewpoint 13/1
  Subsystem16/2(theta) -> Out10/1
  Subsystem13/1(zeta) -> Bias25/1
  Mux13/1 -> Viewpoint 14/1
  Bias27/1 -> Mux13/2
  Subsystem14/2(theta) -> Out6/1
  Sum3/1 -> Display6/1, Mux13/1, Subsystem14/2(x)
  Sum1/1 -> Display5/1, Mux12/1, Subsystem13/2(x)
  Sum2/1 -> Mux14/1, Subsystem15/2(x)
  t/1 -> Subsystem12/1(t), Subsystem13/1(t), Subsystem14/1(t), Subsystem16/1(t), Subsystem15/1(t)
  Product/1 -> Sum/2
  Bias24/1 -> Sum8/2, Bias26/1, Sum/1
  Bias26/1 -> Sum1/1, Sum9/2, Bias28/1
  Round1/1 -> Product1/2
  Divide1/1 -> Round1/1
  Sum9/1 -> Divide1/1
  Product1/1 -> Sum1/2
  Product2/1 -> Sum3/2
  Sum10/1 -> Divide2/1
  Divide2/1 -> Round2/1
  Round2/1 -> Product2/2
  Bias28/1 -> Bias30/1, Sum10/2, Sum3/1
  Bias30/1 -> Sum2/1, Sum11/2, Bias32/1
  Round3/1 -> Product3/2
  Divide3/1 -> Round3/1
  Sum11/1 -> Divide3/1
  Product3/1 -> Sum2/2
  Bias32/1 -> Sum14/2, Sum4/1
  Product6/1 -> Sum4/2
  Sum14/1 -> Divide6/1
  Divide6/1 -> Round6/1
  Round6/1 -> Product6/2
  window width/1 -> Product2/1, Product3/1, Divide6/2, Product6/1, Divide3/2, Divide2/2, Divide1/2, Product1/1, Divide/2, Product/1
  x/1 -> Display11/1, Sum14/1, Sum11/1, Sum10/1, Sum9/1, Sum8/1
  Subsystem13/2(theta) -> Out4/1
  Viewpoint 13/1 -> Out3/1
  Viewpoint 14/1 -> Out5/1

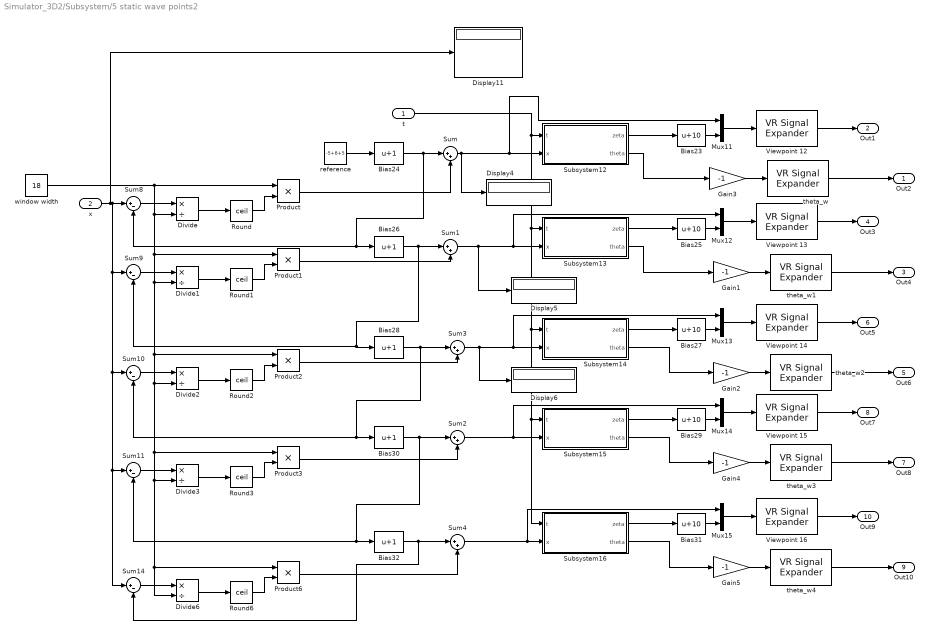
== system Simulator_3D2/Subsystem/5 static wave points2 ==
  t : Inport
  x : Inport  Port=2
  Bias{23,25,27,29,31} (5 alike) : Bias  Bias=10
  Bias{24,26,28,30,32} (5 alike) : Bias  Bias=1
  Display{4..6,11} (4 alike) : Display
  Divide{,1..3,6} (5 alike) : Product  Inputs=*/
  Gain{1..5} (5 alike) : Gain  Gain=-1
  Mux{11..15} (5 alike) : Mux  Inputs=2
  Product{,1..3,6} (5 alike) : Product
  Round{,1..3,6} (5 alike) : Rounding  Operator=ceil
  Subsystem12 : Subsystem
  Subsystem13 : Subsystem
  Subsystem14 : Subsystem
  Subsystem15 : Subsystem
  Subsystem16 : Subsystem
  Sum{,1..4} (5 alike) : Sum  Inputs=|++
  Sum{8..11,14} (5 alike) : Sum  Inputs=|+-
  Viewpoint {12..16} (5 alike) : vrlib/VR Signal Expander  outwidth=3  outidx=[1 2]
      settings: SourceProductName=Simulink 3D Animation  SourceProductBaseCode=VR
  reference : Constant  Value=-5+8+5
  theta_w{,1..4} (5 alike) : vrlib/VR Signal Expander  outwidth=4  outidx=[4]
      settings: SourceProductName=Simulink 3D Animation  SourceProductBaseCode=VR
  window width : Constant  Value=18
  Out2 : Outport
  Out1 : Outport  Port=2
  Out4 : Outport  Port=3
  Out3 : Outport  Port=4
  Out6 : Outport  Port=5
  Out5 : Outport  Port=6
  Out8 : Outport  Port=7
  Out7 : Outport  Port=8
  Out10 : Outport  Port=9
  Out9 : Outport  Port=10
  wires:
  Gain3/1 -> theta_w/1
  Mux12/1 -> Viewpoint 13/1
  theta_w/1 -> Out2/1
  Sum3/1 -> Display6/1, Mux13/1, Subsystem14/2(x)
  theta_w4/1 -> Out10/1
  Viewpoint 12/1 -> Out1/1
  Gain1/1 -> theta_w1/1
  theta_w2/1 -> Out6/1
  Bias29/1 -> Mux14/2
  Subsystem12/2(theta) -> Gain3/1
  Mux11/1 -> Viewpoint 12/1
  theta_w3/1 -> Out8/1
  Gain5/1 -> theta_w4/1
  Subsystem12/1(zeta) -> Bias23/1
  Viewpoint 13/1 -> Out3/1
  Sum/1 -> Display4/1, Subsystem12/2(x), Mux11/1
  Subsystem15/1(zeta) -> Bias29/1
  Subsystem16/1(zeta) -> Bias31/1
  Mux14/1 -> Viewpoint 15/1
  Subsystem14/2(theta) -> Gain2/1
  Bias31/1 -> Mux15/2
  Subsystem14/1(zeta) -> Bias27/1
  Mux15/1 -> Viewpoint 16/1
  Bias23/1 -> Mux11/2
  Viewpoint 16/1 -> Out9/1
  Viewpoint 14/1 -> Out5/1
  Subsystem13/1(zeta) -> Bias25/1
  Mux13/1 -> Viewpoint 14/1
  Bias25/1 -> Mux12/2
  Bias27/1 -> Mux13/2
  Subsystem15/2(theta) -> Gain4/1
  Sum4/1 -> Subsystem16/2(x), Mux15/1
  Sum1/1 -> Display5/1, Mux12/1, Subsystem13/2(x)
  Sum2/1 -> Mux14/1, Subsystem15/2(x)
  Viewpoint 15/1 -> Out7/1
  Subsystem16/2(theta) -> Gain5/1
  theta_w1/1 -> Out4/1
  Gain4/1 -> theta_w3/1
  Gain2/1 -> theta_w2/1
  Subsystem13/2(theta) -> Gain1/1
  reference/1 -> Bias24/1
  Sum8/1 -> Divide/1
  Divide/1 -> Round/1
  Round/1 -> Product/2
  t/1 -> Subsystem12/1(t), Subsystem13/1(t), Subsystem14/1(t), Subsystem16/1(t), Subsystem15/1(t)
  Product/1 -> Sum/2
  Bias24/1 -> Sum8/2, Bias26/1, Sum/1
  Bias26/1 -> Sum1/1, Sum9/2, Bias28/1
  Round1/1 -> Product1/2
  Divide1/1 -> Round1/1
  Sum9/1 -> Divide1/1
  Product1/1 -> Sum1/2
  Product2/1 -> Sum3/2
  Sum10/1 -> Divide2/1
  Divide2/1 -> Round2/1
  Round2/1 -> Product2/2
  Bias28/1 -> Bias30/1, Sum10/2, Sum3/1
  Bias30/1 -> Sum2/1, Sum11/2, Bias32/1
  Round3/1 -> Product3/2
  Divide3/1 -> Round3/1
  Sum11/1 -> Divide3/1
  Product3/1 -> Sum2/2
  Bias32/1 -> Sum14/2, Sum4/1
  Product6/1 -> Sum4/2
  Sum14/1 -> Divide6/1
  Divide6/1 -> Round6/1
  Round6/1 -> Product6/2
  window width/1 -> Product2/1, Product3/1, Divide6/2, Product6/1, Divide3/2, Divide2/2, Divide1/2, Product1/1, Divide/2, Product/1
  x/1 -> Display11/1, Sum14/1, Sum11/1, Sum10/1, Sum9/1, Sum8/1

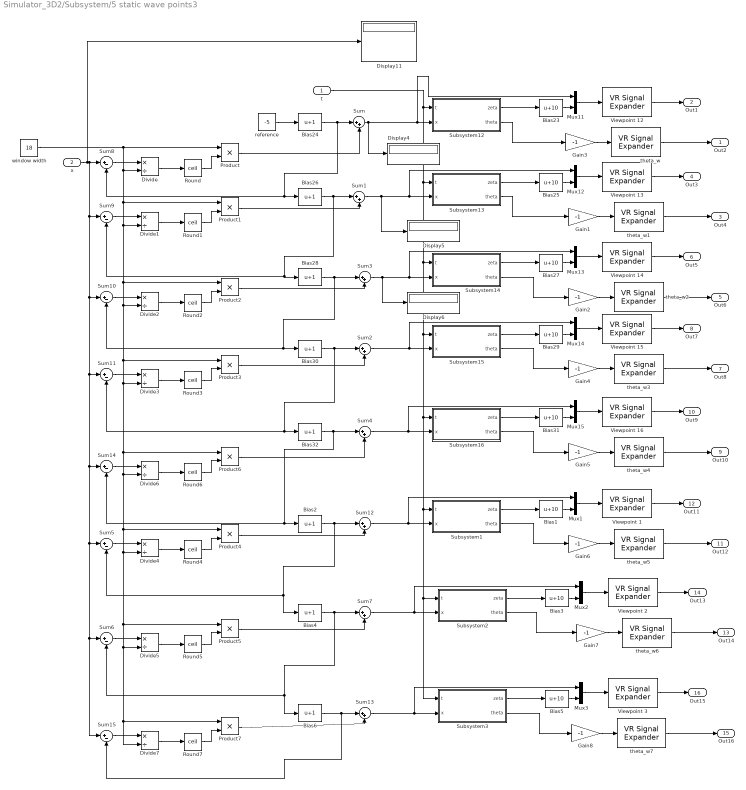
== system Simulator_3D2/Subsystem/5 static wave points3 ==
  t : Inport
  x : Inport  Port=2
  Bias{1,3,5,23,25,27,29,31} (8 alike) : Bias  Bias=10
  Bias{2,4,6,24,26,28,30,32} (8 alike) : Bias  Bias=1
  Display{4..6,11} (4 alike) : Display
  Divide{,1..7} (8 alike) : Product  Inputs=*/
  Gain{1..8} (8 alike) : Gain  Gain=-1
  Mux{1..3,11..15} (8 alike) : Mux  Inputs=2
  Product{,1..7} (8 alike) : Product
  Round{,1..7} (8 alike) : Rounding  Operator=ceil
  Subsystem1 : Subsystem
  Subsystem12 : Subsystem
  Subsystem13 : Subsystem
  Subsystem14 : Subsystem
  Subsystem15 : Subsystem
  Subsystem16 : Subsystem
  Subsystem2 : Subsystem
  Subsystem3 : Subsystem
  Sum{,1..4,7,12..13} (8 alike) : Sum  Inputs=|++
  Sum{5..6,8..11,14..15} (8 alike) : Sum  Inputs=|+-
  Viewpoint {1..3,12..16} (8 alike) : vrlib/VR Signal Expander  outwidth=3  outidx=[1 2]
      settings: SourceProductName=Simulink 3D Animation  SourceProductBaseCode=VR
  reference : Constant  Value=-5
  theta_w{,1..7} (8 alike) : vrlib/VR Signal Expander  outwidth=4  outidx=[4]
      settings: SourceProductName=Simulink 3D Animation  SourceProductBaseCode=VR
  window width : Constant  Value=18
  Out2 : Outport
  Out1 : Outport  Port=2
  Out4 : Outport  Port=3
  Out3 : Outport  Port=4
  Out6 : Outport  Port=5
  Out5 : Outport  Port=6
  Out8 : Outport  Port=7
  Out7 : Outport  Port=8
  Out10 : Outport  Port=9
  Out9 : Outport  Port=10
  Out12 : Outport  Port=11
  Out11 : Outport  Port=12
  Out14 : Outport  Port=13
  Out13 : Outport  Port=14
  Out16 : Outport  Port=15
  Out15 : Outport  Port=16
  wires:
  reference/1 -> Bias24/1
  Sum8/1 -> Divide/1
  Divide/1 -> Round/1
  Round/1 -> Product/2
  Subsystem15/1(zeta) -> Bias29/1
  Viewpoint 15/1 -> Out7/1
  Subsystem12/1(zeta) -> Bias23/1
  Viewpoint 12/1 -> Out1/1
  Mux14/1 -> Viewpoint 15/1
  Sum/1 -> Display4/1, Mux11/1, Subsystem12/2(x)
  Bias29/1 -> Mux14/2
  Subsystem16/1(zeta) -> Bias31/1
  Subsystem12/2(theta) -> Gain3/1
  Sum4/1 -> Mux15/1, Subsystem16/2(x)
  Viewpoint 16/1 -> Out9/1
  Bias31/1 -> Mux15/2
  Mux15/1 -> Viewpoint 16/1
  Bias25/1 -> Mux12/2
  Subsystem14/1(zeta) -> Bias27/1
  Mux11/1 -> Viewpoint 12/1
  Bias23/1 -> Mux11/2
  Mux12/1 -> Viewpoint 13/1
  Subsystem13/1(zeta) -> Bias25/1
  Mux13/1 -> Viewpoint 14/1
  Bias27/1 -> Mux13/2
  Sum3/1 -> Display6/1, Mux13/1, Subsystem14/2(x)
  Sum1/1 -> Display5/1, Mux12/1, Subsystem13/2(x)
  Sum2/1 -> Mux14/1, Subsystem15/2(x)
  Mux1/1 -> Viewpoint 1/1
  Bias1/1 -> Mux1/2
  Viewpoint 1/1 -> Out11/1
  Sum12/1 -> Subsystem1/2(x), Mux1/1
  Subsystem1/1(zeta) -> Bias1/1
  Subsystem2/1(zeta) -> Bias3/1
  Sum7/1 -> Mux2/1, Subsystem2/2(x)
  Viewpoint 2/1 -> Out13/1
  Bias3/1 -> Mux2/2
  Mux2/1 -> Viewpoint 2/1
  Mux3/1 -> Viewpoint 3/1
  Bias5/1 -> Mux3/2
  Viewpoint 3/1 -> Out15/1
  Sum13/1 -> Subsystem3/2(x), Mux3/1
  Subsystem3/1(zeta) -> Bias5/1
  t/1 -> Subsystem12/1(t), Subsystem13/1(t), Subsystem14/1(t), Subsystem3/1(t), Subsystem2/1(t), Subsystem1/1(t), Subsystem16/1(t), Subsystem15/1(t)
  Product/1 -> Sum/2
  Bias24/1 -> Sum8/2, Bias26/1, Sum/1
  Bias26/1 -> Sum1/1, Sum9/2, Bias28/1
  Round1/1 -> Product1/2
  Divide1/1 -> Round1/1
  Sum9/1 -> Divide1/1
  Product1/1 -> Sum1/2
  Product2/1 -> Sum3/2
  Sum10/1 -> Divide2/1
  Divide2/1 -> Round2/1
  Round2/1 -> Product2/2
  Bias28/1 -> Bias30/1, Sum10/2, Sum3/1
  Bias30/1 -> Sum2/1, Sum11/2, Bias32/1
  Round3/1 -> Product3/2
  Divide3/1 -> Round3/1
  Sum11/1 -> Divide3/1
  Product3/1 -> Sum2/2
  Product4/1 -> Sum12/2
  Product5/1 -> Sum7/2
  Sum5/1 -> Divide4/1
  Divide4/1 -> Round4/1
  Round4/1 -> Product4/2
  Bias32/1 -> Sum14/2, Bias2/1, Sum4/1
  Bias4/1 -> Sum7/1, Sum6/2, Bias6/1
  Bias2/1 -> Bias4/1, Sum5/2, Sum12/1
  Round5/1 -> Product5/2
  Divide5/1 -> Round5/1
  Sum6/1 -> Divide5/1
  Product6/1 -> Sum4/2
  Sum14/1 -> Divide6/1
  Divide6/1 -> Round6/1
  Round6/1 -> Product6/2
  Sum15/1 -> Divide7/1
  Divide7/1 -> Round7/1
  Round7/1 -> Product7/2
  Bias6/1 -> Sum15/2, Sum13/1
  window width/1 -> Product2/1, Product3/1, Product5/1, Divide7/2, Product7/1, Divide5/2, Divide4/2, Product4/1, Divide6/2, Product6/1, Divide3/2, Divide2/2, Divide1/2, Product1/1, Divide/2, Product/1
  Product7/1 -> Sum13/2
  x/1 -> Display11/1, Sum15/1, Sum6/1, Sum5/1, Sum14/1, Sum11/1, Sum10/1, Sum9/1, Sum8/1
  Viewpoint 13/1 -> Out3/1
  Viewpoint 14/1 -> Out5/1
  Gain3/1 -> theta_w/1
  theta_w/1 -> Out2/1
  theta_w1/1 -> Out4/1
  Gain1/1 -> theta_w1/1
  Subsystem13/2(theta) -> Gain1/1
  Gain2/1 -> theta_w2/1
  theta_w2/1 -> Out6/1
  Subsystem14/2(theta) -> Gain2/1
  Gain4/1 -> theta_w3/1
  theta_w3/1 -> Out8/1
  Subsystem15/2(theta) -> Gain4/1
  Subsystem16/2(theta) -> Gain5/1
  theta_w4/1 -> Out10/1
  Gain5/1 -> theta_w4/1
  Subsystem1/2(theta) -> Gain6/1
  theta_w5/1 -> Out12/1
  Gain6/1 -> theta_w5/1
  Subsystem2/2(theta) -> Gain7/1
  theta_w6/1 -> Out14/1
  Gain7/1 -> theta_w6/1
  Subsystem3/2(theta) -> Gain8/1
  theta_w7/1 -> Out16/1
  Gain8/1 -> theta_w7/1

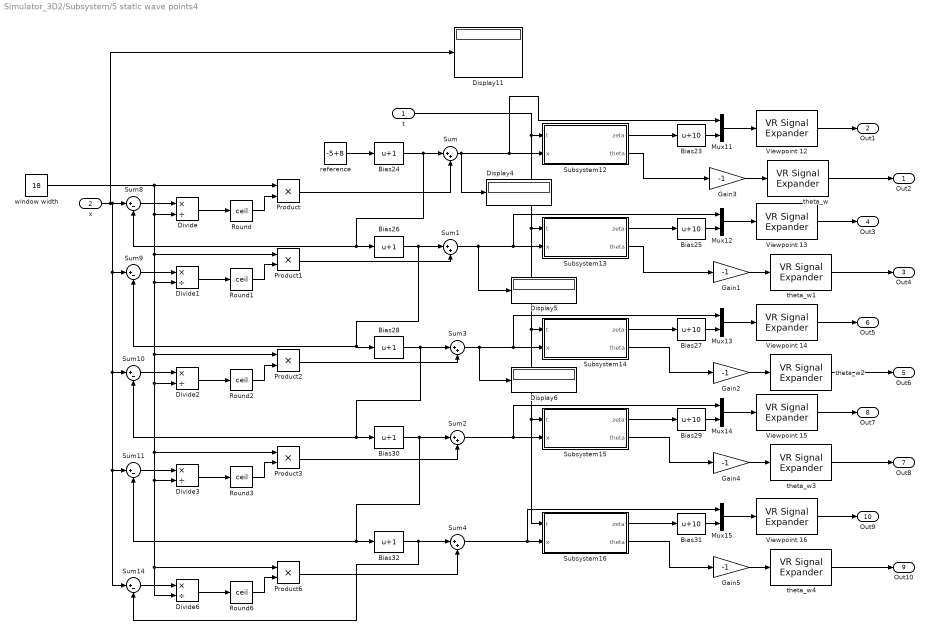
== system Simulator_3D2/Subsystem/5 static wave points4 ==
  t : Inport
  x : Inport  Port=2
  Bias{23,25,27,29,31} (5 alike) : Bias  Bias=10
  Bias{24,26,28,30,32} (5 alike) : Bias  Bias=1
  Display{4..6,11} (4 alike) : Display
  Divide{,1..3,6} (5 alike) : Product  Inputs=*/
  Gain{1..5} (5 alike) : Gain  Gain=-1
  Mux{11..15} (5 alike) : Mux  Inputs=2
  Product{,1..3,6} (5 alike) : Product
  Round{,1..3,6} (5 alike) : Rounding  Operator=ceil
  Subsystem12 : Subsystem
  Subsystem13 : Subsystem
  Subsystem14 : Subsystem
  Subsystem15 : Subsystem
  Subsystem16 : Subsystem
  Sum{,1..4} (5 alike) : Sum  Inputs=|++
  Sum{8..11,14} (5 alike) : Sum  Inputs=|+-
  Viewpoint {12..16} (5 alike) : vrlib/VR Signal Expander  outwidth=3  outidx=[1 2]
      settings: SourceProductName=Simulink 3D Animation  SourceProductBaseCode=VR
  reference : Constant  Value=-5+8
  theta_w{,1..4} (5 alike) : vrlib/VR Signal Expander  outwidth=4  outidx=[4]
      settings: SourceProductName=Simulink 3D Animation  SourceProductBaseCode=VR
  window width : Constant  Value=18
  Out2 : Outport
  Out1 : Outport  Port=2
  Out4 : Outport  Port=3
  Out3 : Outport  Port=4
  Out6 : Outport  Port=5
  Out5 : Outport  Port=6
  Out8 : Outport  Port=7
  Out7 : Outport  Port=8
  Out10 : Outport  Port=9
  Out9 : Outport  Port=10
  wires:
  x/1 -> Sum8/1, Sum9/1, Sum10/1, Sum11/1, Sum14/1, Display11/1
  window width/1 -> Product/1, Divide/2, Product1/1, Divide1/2, Divide2/2, Divide3/2, Product6/1, Divide6/2, Product3/1, Product2/1
  Round6/1 -> Product6/2
  Divide6/1 -> Round6/1
  Sum14/1 -> Divide6/1
  Product6/1 -> Sum4/2
  Bias32/1 -> Sum4/1, Sum14/2
  Product3/1 -> Sum2/2
  Sum11/1 -> Divide3/1
  Divide3/1 -> Round3/1
  Round3/1 -> Product3/2
  Bias30/1 -> Bias32/1, Sum11/2, Sum2/1
  Bias28/1 -> Sum3/1, Sum10/2, Bias30/1
  Round2/1 -> Product2/2
  Divide2/1 -> Round2/1
  Sum10/1 -> Divide2/1
  Product2/1 -> Sum3/2
  Product1/1 -> Sum1/2
  Sum9/1 -> Divide1/1
  Divide1/1 -> Round1/1
  Round1/1 -> Product1/2
  Bias26/1 -> Bias28/1, Sum9/2, Sum1/1
  Bias24/1 -> Sum/1, Bias26/1, Sum8/2
  Product/1 -> Sum/2
  t/1 -> Subsystem15/1(t), Subsystem16/1(t), Subsystem14/1(t), Subsystem13/1(t), Subsystem12/1(t)
  Round/1 -> Product/2
  Divide/1 -> Round/1
  Sum8/1 -> Divide/1
  reference/1 -> Bias24/1
  Subsystem13/2(theta) -> Gain1/1
  Gain2/1 -> theta_w2/1
  Gain4/1 -> theta_w3/1
  theta_w1/1 -> Out4/1
  Subsystem16/2(theta) -> Gain5/1
  Viewpoint 15/1 -> Out7/1
  Sum2/1 -> Subsystem15/2(x), Mux14/1
  Sum1/1 -> Subsystem13/2(x), Mux12/1, Display5/1
  Sum4/1 -> Mux15/1, Subsystem16/2(x)
  Subsystem15/2(theta) -> Gain4/1
  Bias27/1 -> Mux13/2
  Bias25/1 -> Mux12/2
  Mux13/1 -> Viewpoint 14/1
  Subsystem13/1(zeta) -> Bias25/1
  Viewpoint 14/1 -> Out5/1
  Viewpoint 16/1 -> Out9/1
  Bias23/1 -> Mux11/2
  Mux15/1 -> Viewpoint 16/1
  Subsystem14/1(zeta) -> Bias27/1
  Bias31/1 -> Mux15/2
  Subsystem14/2(theta) -> Gain2/1
  Mux14/1 -> Viewpoint 15/1
  Subsystem16/1(zeta) -> Bias31/1
  Subsystem15/1(zeta) -> Bias29/1
  Sum/1 -> Mux11/1, Subsystem12/2(x), Display4/1
  Viewpoint 13/1 -> Out3/1
  Subsystem12/1(zeta) -> Bias23/1
  Gain5/1 -> theta_w4/1
  theta_w3/1 -> Out8/1
  Mux11/1 -> Viewpoint 12/1
  Subsystem12/2(theta) -> Gain3/1
  Bias29/1 -> Mux14/2
  theta_w2/1 -> Out6/1
  Gain1/1 -> theta_w1/1
  Viewpoint 12/1 -> Out1/1
  theta_w4/1 -> Out10/1
  Sum3/1 -> Subsystem14/2(x), Mux13/1, Display6/1
  theta_w/1 -> Out2/1
  Mux12/1 -> Viewpoint 13/1
  Gain3/1 -> theta_w/1

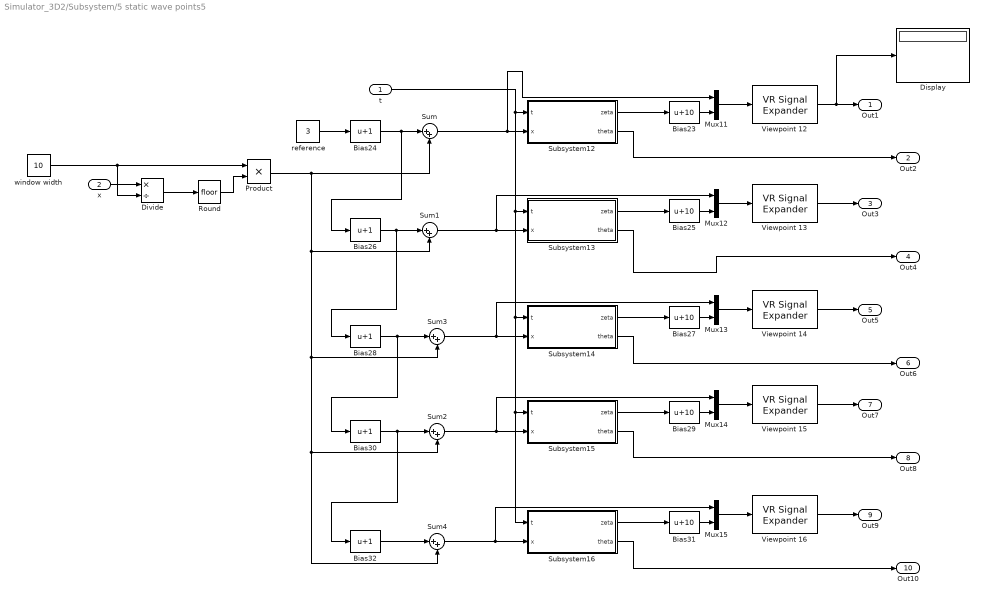
== system Simulator_3D2/Subsystem/5 static wave points5 ==
  t : Inport
  x : Inport  Port=2
  Bias{23,25,27,29,31} (5 alike) : Bias  Bias=10
  Bias{24,26,28,30,32} (5 alike) : Bias  Bias=1
  Display : Display
  Divide : Product  Inputs=*/
  Mux{11..15} (5 alike) : Mux  Inputs=2
  Product : Product
  Round : Rounding
  Subsystem12 : Subsystem
  Subsystem13 : Subsystem
  Subsystem14 : Subsystem
  Subsystem15 : Subsystem
  Subsystem16 : Subsystem
  Sum{,1..4} (5 alike) : Sum  Inputs=|++
  Viewpoint {12..16} (5 alike) : vrlib/VR Signal Expander  outwidth=3  outidx=[1 2]
      settings: SourceProductName=Simulink 3D Animation  SourceProductBaseCode=VR
  reference : Constant  Value=3
  window width : Constant  Value=10
  Out1 : Outport
  Out2 : Outport  Port=2
  Out3 : Outport  Port=3
  Out4 : Outport  Port=4
  Out5 : Outport  Port=5
  Out6 : Outport  Port=6
  Out7 : Outport  Port=7
  Out8 : Outport  Port=8
  Out9 : Outport  Port=9
  Out10 : Outport  Port=10
  wires:
  Viewpoint 14/1 -> Out5/1
  Viewpoint 13/1 -> Out3/1
  Bias28/1 -> Sum3/1, Bias30/1
  Bias30/1 -> Sum2/1, Bias32/1
  Bias32/1 -> Sum4/1
  Bias26/1 -> Sum1/1, Bias28/1
  Product/1 -> Sum/2, Sum1/2, Sum3/2, Sum2/2, Sum4/2
  reference/1 -> Bias24/1
  Bias24/1 -> Sum/1, Bias26/1
  window width/1 -> Product/1, Divide/2
  x/1 -> Divide/1
  Divide/1 -> Round/1
  Round/1 -> Product/2
  t/1 -> Subsystem12/1(t), Subsystem13/1(t), Subsystem14/1(t), Subsystem16/1(t), Subsystem15/1(t)
  Subsystem15/1(zeta) -> Bias29/1
  Viewpoint 15/1 -> Out7/1
  Subsystem12/1(zeta) -> Bias23/1
  Viewpoint 12/1 -> Out1/1, Display/1
  Mux14/1 -> Viewpoint 15/1
  Sum/1 -> Mux11/1, Subsystem12/2(x)
  Bias29/1 -> Mux14/2
  Subsystem16/1(zeta) -> Bias31/1
  Subsystem12/2(theta) -> Out2/1
  Sum4/1 -> Mux15/1, Subsystem16/2(x)
  Viewpoint 16/1 -> Out9/1
  Bias31/1 -> Mux15/2
  Mux15/1 -> Viewpoint 16/1
  Subsystem15/2(theta) -> Out8/1
  Bias25/1 -> Mux12/2
  Subsystem14/1(zeta) -> Bias27/1
  Mux11/1 -> Viewpoint 12/1
  Bias23/1 -> Mux11/2
  Mux12/1 -> Viewpoint 13/1
  Subsystem16/2(theta) -> Out10/1
  Subsystem13/1(zeta) -> Bias25/1
  Mux13/1 -> Viewpoint 14/1
  Bias27/1 -> Mux13/2
  Subsystem13/2(theta) -> Out4/1
  Subsystem14/2(theta) -> Out6/1
  Sum3/1 -> Mux13/1, Subsystem14/2(x)
  Sum1/1 -> Mux12/1, Subsystem13/2(x)
  Sum2/1 -> Mux14/1, Subsystem15/2(x)

== system Simulator_3D2/Subsystem/5 static wave points6 ==
  t : Inport
  x : Inport  Port=2
  Bias{23,25,27,29,31} (5 alike) : Bias  Bias=10
  Bias{24,26,28,30,32} (5 alike) : Bias  Bias=1
  Display : Display
  Divide : Product  Inputs=*/
  Mux{11..15} (5 alike) : Mux  Inputs=2
  Product : Product
  Round : Rounding
  Subsystem12 : Subsystem
  Subsystem13 : Subsystem
  Subsystem14 : Subsystem
  Subsystem15 : Subsystem
  Subsystem16 : Subsystem
  Sum{,1..4} (5 alike) : Sum  Inputs=|++
  Viewpoint {12..16} (5 alike) : vrlib/VR Signal Expander  outwidth=3  outidx=[1 2]
      settings: SourceProductName=Simulink 3D Animation  SourceProductBaseCode=VR
  reference : Constant  Value=5+3
  window width : Constant  Value=10
  Out1 : Outport
  Out2 : Outport  Port=2
  Out3 : Outport  Port=3
  Out4 : Outport  Port=4
  Out5 : Outport  Port=5
  Out6 : Outport  Port=6
  Out7 : Outport  Port=7
  Out8 : Outport  Port=8
  Out9 : Outport  Port=9
  Out10 : Outport  Port=10
  wires:
  Sum2/1 -> Subsystem15/2(x), Mux14/1
  Sum1/1 -> Subsystem13/2(x), Mux12/1
  Sum3/1 -> Subsystem14/2(x), Mux13/1
  Subsystem14/2(theta) -> Out6/1
  Subsystem13/2(theta) -> Out4/1
  Bias27/1 -> Mux13/2
  Mux13/1 -> Viewpoint 14/1
  Subsystem13/1(zeta) -> Bias25/1
  Subsystem16/2(theta) -> Out10/1
  Mux12/1 -> Viewpoint 13/1
  Bias23/1 -> Mux11/2
  Mux11/1 -> Viewpoint 12/1
  Subsystem14/1(zeta) -> Bias27/1
  Bias25/1 -> Mux12/2
  Subsystem15/2(theta) -> Out8/1
  Mux15/1 -> Viewpoint 16/1
  Bias31/1 -> Mux15/2
  Viewpoint 16/1 -> Out9/1
  Sum4/1 -> Subsystem16/2(x), Mux15/1
  Subsystem12/2(theta) -> Out2/1
  Subsystem16/1(zeta) -> Bias31/1
  Bias29/1 -> Mux14/2
  Sum/1 -> Subsystem12/2(x), Mux11/1
  Mux14/1 -> Viewpoint 15/1
  Viewpoint 12/1 -> Display/1, Out1/1
  Subsystem12/1(zeta) -> Bias23/1
  Viewpoint 15/1 -> Out7/1
  Subsystem15/1(zeta) -> Bias29/1
  t/1 -> Subsystem15/1(t), Subsystem16/1(t), Subsystem14/1(t), Subsystem13/1(t), Subsystem12/1(t)
  Round/1 -> Product/2
  Divide/1 -> Round/1
  x/1 -> Divide/1
  window width/1 -> Divide/2, Product/1
  Bias24/1 -> Bias26/1, Sum/1
  reference/1 -> Bias24/1
  Product/1 -> Sum4/2, Sum2/2, Sum3/2, Sum1/2, Sum/2
  Bias26/1 -> Bias28/1, Sum1/1
  Bias32/1 -> Sum4/1
  Bias30/1 -> Bias32/1, Sum2/1
  Bias28/1 -> Bias30/1, Sum3/1
  Viewpoint 13/1 -> Out3/1
  Viewpoint 14/1 -> Out5/1
